simulink model "sampleModel1936_sub_sub_sub"  (R2023a)
settings: Solver=VariableStepAuto  StartTime=0.0  StopTime=10.0  RelTol=1e-3
libraries: hdlsllib x7
settings Model: Creator=user1  LastModifiedBy=user1
settings OptimizationCC: BlockReduction=off  ConditionallyExecuteInputs=off

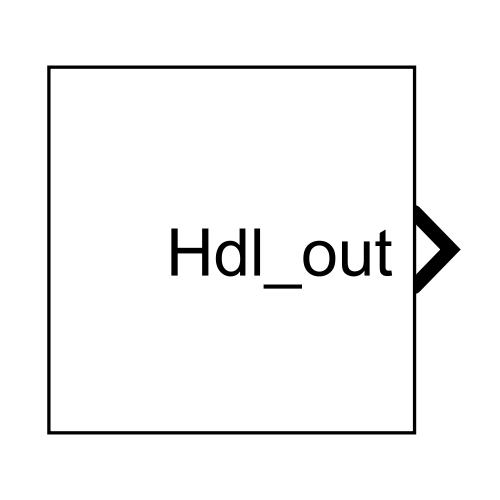
[thumbnail: Simulink's stored preview of the top-level diagram]
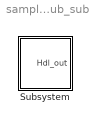
== system sampleModel1936_sub_sub_sub ==
  Subsystem : Subsystem

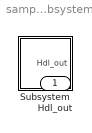
== system sampleModel1936_sub_sub_sub/Subsystem ==
  Subsystem : Subsystem
  Hdl_out : Outport  OutDataTypeStr=uint8

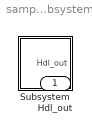
== system sampleModel1936_sub_sub_sub/Subsystem/Subsystem ==
  Subsystem : Subsystem
  Hdl_out : Outport  OutDataTypeStr=uint8

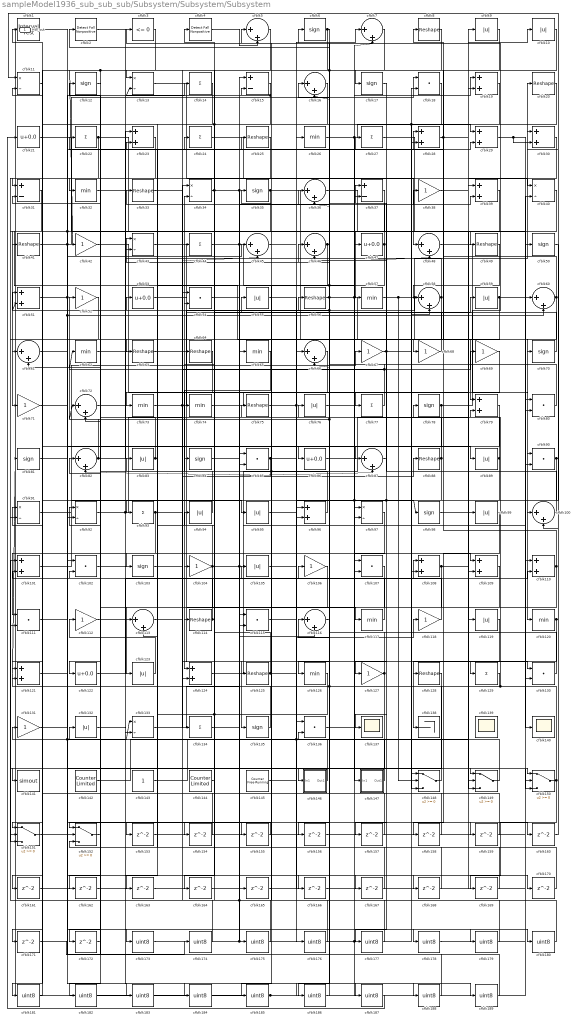
== system sampleModel1936_sub_sub_sub/Subsystem/Subsystem/Subsystem ==
  cfblk1 : hdlsllib/Logic and Bit Operations/Interval Test  IntervalClosedRight=on  uplimit=0.5  IntervalClosedLeft=on  lowlimit=-0.5  OutDataTypeStr=uint8
  cfblk{9..10,55,59,76,83,89,94..95,99,105,119,123,132} (14 alike) : Abs  OutDataTypeStr=uint8  SaturateOnIntegerOverflow=off
  cfblk{5,7,16,36,45..46,48,58,60..61,66,72,82,87,100,113,116} (17 alike) : Sum  Inputs=|++  OutDataTypeStr=uint8
  cfblk{19,23,28..30,39,51,79,96,101,108..110,121,124} (15 alike) : Sum  OutDataTypeStr=uint8
  cfblk{18,54,80,85,90,102,107,111,115,130,136} (11 alike) : DotProduct  OutDataTypeStr=uint8
  cfblk{6,12,17,35,50,70,78,81,84,98,103,135} (12 alike) : Signum
  cfblk{38,42,52,67..69,71,104,106,112,118,127,131} (13 alike) : Gain  OutDataTypeStr=uint8
  cfblk{11,13,34,40,43,91..92,97,133} (9 alike) : Product  Inputs=*/  OutDataTypeStr=uint8  RndMeth=Zero  SaturateOnIntegerOverflow=on
  cfblk{8,20,25,33,41,49,56,63..64,75,88,114,125,128} (14 alike) : Reshape
  cfblk{26,32,57,62,65,73..74,117,120,126} (10 alike) : MinMax  OutDataTypeStr=uint8
  cfblk{21,47,53,86,122} (5 alike) : Bias  Bias=0.0  SaturateOnIntegerOverflow=off
  cfblk{14,22,24,27,44,77,93,129,134} (9 alike) : Sum  Inputs=+  OutDataTypeStr=uint8
  cfblk137 : Scope
  cfblk138 : Terminator
  cfblk139 : Scope
      settings: Floating=on
  cfblk140 : Scope
  cfblk141 : ToWorkspace  VariableName=simout  SaveFormat=Timeseries  SampleTime=-1
  cfblk142 : hdlsllib/Sources/Counter Limited  uplimit=7  tsamp=-1
  cfblk143 : Constant  OutDataTypeStr=uint8  SampleTime=-1
  cfblk144 : hdlsllib/Sources/Counter Limited  uplimit=7  tsamp=-1
  cfblk145 : hdlsllib/Sources/Counter Free-Running  NumBits=16  tsamp=-1
  cfblk146 : Subsystem
      settings: LibrarySourceBlock=|
      | hdlsllib/Ports &
      | Subsystems/Subsystem
  cfblk147 : Subsystem
      settings: LibrarySourceBlock=|
      | hdlsllib/Ports &
      | Subsystems/Subsystem
  cfblk{148..152} (5 alike) : Switch  OutDataTypeStr=uint8  SaturateOnIntegerOverflow=off  InputSameDT=off
  cfblk15 : Sum  Inputs=+-  OutDataTypeStr=uint8
  cfblk{153..172} (20 alike) : Delay  SampleTime=1
  cfblk{173..189} (17 alike) : DataTypeConversion  OutDataTypeStr=uint8  SaturateOnIntegerOverflow=off  RndMeth=Floor
  cfblk2 : hdlsllib/Logic and Bit Operations/Detect Fall Nonpositive  vinit=0  OutDataTypeStr=uint8
  cfblk3 : hdlsllib/Logic and Bit Operations/Compare To Zero  relop=<=  OutDataTypeStr=uint8
  cfblk31 : Sum  Inputs=+-  OutDataTypeStr=uint8
  cfblk37 : Sum  Inputs=+-  OutDataTypeStr=uint8
  cfblk4 : hdlsllib/Logic and Bit Operations/Detect Fall Nonpositive  vinit=0  OutDataTypeStr=uint8
  Hdl_out : Outport  OutDataTypeStr=uint8
  wires:
  cfblk58/1 -> cfblk151/2, cfblk43/1
  cfblk74/1 -> cfblk77/1
  cfblk49/1 -> cfblk55/1
  cfblk78/1 -> cfblk141/1, cfblk6/1
  cfblk150/1 -> cfblk169/1, cfblk79/2, cfblk36/1, cfblk81/1
  cfblk65/1 -> cfblk124/1
  cfblk82/1 -> cfblk25/1, cfblk52/1
  cfblk97/1 -> cfblk103/1
  cfblk41/1 -> cfblk150/1, cfblk18/1
  cfblk31/1 -> cfblk79/1
  cfblk3/1 -> cfblk32/1, cfblk42/1
  cfblk101/1 -> cfblk67/1
  cfblk53/1 -> cfblk135/1
  cfblk88/1 -> cfblk171/1, cfblk53/1
  cfblk108/1 -> cfblk150/2, cfblk123/1
  cfblk70/1 -> cfblk4/1
  cfblk130/1 -> cfblk72/1, cfblk51/2, cfblk36/2
  cfblk7/1 -> cfblk124/2
  cfblk13/1 -> cfblk97/1
  cfblk48/1 -> cfblk120/1
  cfblk9/1 -> cfblk68/1
  cfblk94/1 -> cfblk34/2
  cfblk93/1 -> cfblk88/1, cfblk111/1
  cfblk43/1 -> cfblk117/1
  cfblk5/1 -> cfblk121/1
  cfblk118/1 -> cfblk35/1
  cfblk63/1 -> cfblk59/1
  cfblk125/1 -> cfblk118/1, cfblk24/1
  cfblk26/1 -> cfblk48/2, cfblk29/1
  cfblk33/1 -> cfblk89/1
  cfblk126/1 -> cfblk164/1, cfblk163/1
  cfblk46/1 -> cfblk155/1, cfblk16/1
  cfblk35/1 -> cfblk148/1, cfblk111/2, cfblk92/2
  cfblk51/1 -> cfblk159/1, cfblk14/1
  cfblk83/1 -> cfblk31/2, cfblk113/1
  cfblk56/1 -> cfblk16/2, cfblk7/2, cfblk90/1
  cfblk22/1 -> cfblk91/2, cfblk57/1
  cfblk15/1 -> cfblk181/1, cfblk13/2
  cfblk64/1 -> cfblk73/1
  cfblk40/1 -> cfblk71/1
  cfblk96/1 -> cfblk61/2, cfblk15/2
  cfblk131/1 -> cfblk180/1
  cfblk76/1 -> cfblk109/1
  cfblk129/1 -> cfblk121/2
  cfblk6/1 -> cfblk13/1, cfblk126/1
  cfblk1/1 -> cfblk173/1
  cfblk114/1 -> cfblk12/1, cfblk84/1
  cfblk148/1 -> cfblk51/1, cfblk76/1
  cfblk8/1 -> cfblk17/1
  cfblk66/1 -> cfblk96/2
  cfblk34/1 -> cfblk154/1, cfblk87/2, cfblk29/2
  cfblk47/1 -> cfblk2/1, cfblk63/1, cfblk66/2
  cfblk68/1 -> cfblk5/1
  cfblk30/1 -> cfblk104/1
  cfblk147/1(Out1) -> cfblk136/2
  cfblk90/1 -> cfblk177/1, cfblk11/1
  cfblk80/1 -> cfblk33/1
  cfblk98/1 -> cfblk109/2
  cfblk115/1 -> cfblk108/1
  cfblk133/1 -> cfblk65/1
  cfblk24/1 -> cfblk48/1
  cfblk87/1 -> cfblk37/1
  cfblk59/1 -> cfblk87/1, cfblk60/1
  cfblk127/1 -> cfblk151/3, cfblk3/1
  cfblk73/1 -> cfblk45/2, cfblk20/1
  cfblk142/1 -> cfblk9/1
  cfblk21/1 -> cfblk110/1
  cfblk79/1 -> cfblk113/2
  cfblk62/1 -> cfblk134/1
  cfblk20/1 -> cfblk127/1
  cfblk28/1 -> cfblk58/1, cfblk10/1
  cfblk39/1 -> cfblk122/1
  cfblk89/1 -> cfblk75/1, cfblk115/2, cfblk137/1
  cfblk135/1 -> cfblk82/1
  cfblk60/1 -> cfblk70/1, cfblk22/1
  cfblk95/1 -> cfblk149/1
  cfblk110/1 -> cfblk156/1, cfblk8/1
  cfblk103/1 -> cfblk129/1
  cfblk50/1 -> cfblk100/1
  cfblk120/1 -> cfblk149/3, cfblk30/1
  cfblk117/1 -> cfblk11/2
  cfblk71/1 -> cfblk85/2
  cfblk143/1 -> cfblk28/2, cfblk26/1
  cfblk122/1 -> cfblk110/2
  cfblk119/1 -> cfblk138/1
  cfblk72/1 -> cfblk23/1
  cfblk23/1 -> cfblk152/2
  cfblk11/1 -> cfblk31/1
  cfblk151/1 -> cfblk133/1, cfblk27/1
  cfblk146/1(Out1) -> cfblk91/1
  cfblk29/1 -> cfblk30/2, cfblk140/1
  cfblk136/1 -> cfblk19/1
  cfblk45/1 -> cfblk7/1
  cfblk57/1 -> cfblk148/2, cfblk40/2, cfblk119/1
  cfblk37/1 -> cfblk146/1(In1)
  cfblk67/1 -> cfblk37/2, cfblk130/1
  cfblk144/1 -> cfblk64/1
  cfblk124/1 -> cfblk39/1
  cfblk27/1 -> cfblk99/1
  cfblk84/1 -> cfblk116/2
  cfblk123/1 -> cfblk112/1
  cfblk36/1 -> cfblk49/1
  cfblk100/1 -> cfblk46/2
  cfblk14/1 -> cfblk41/1
  cfblk19/1 -> cfblk108/2, cfblk151/1, cfblk114/1
  cfblk85/1 -> cfblk28/1, cfblk82/2
  cfblk44/1 -> cfblk39/2, cfblk147/1(In1)
  cfblk91/1 -> cfblk95/1
  cfblk99/1 -> cfblk128/1
  cfblk4/1 -> cfblk5/2
  cfblk111/1 -> cfblk60/2, cfblk45/1
  cfblk86/1 -> cfblk78/1
  cfblk75/1 -> cfblk38/1, cfblk97/2, cfblk98/1
  cfblk152/1 -> cfblk92/1
  cfblk113/1 -> cfblk69/1
  cfblk18/1 -> cfblk61/1
  cfblk92/1 -> cfblk150/3, cfblk44/1
  cfblk38/1 -> cfblk40/1
  cfblk104/1 -> cfblk133/2, cfblk83/1, cfblk148/3, cfblk50/1
  cfblk77/1 -> cfblk43/2, cfblk62/1
  cfblk10/1 -> cfblk74/1, cfblk86/1
  cfblk116/1 -> cfblk56/1
  cfblk42/1 -> cfblk149/2
  cfblk16/1 -> cfblk93/1
  cfblk149/1 -> cfblk132/1
  cfblk69/1 -> cfblk153/1
  cfblk153/1 -> cfblk90/2
  cfblk154/1 -> cfblk101/2
  cfblk155/1 -> cfblk152/1
  cfblk156/1 -> cfblk46/1
  cfblk17/1 -> cfblk157/1
  cfblk157/1 -> cfblk34/1
  cfblk109/1 -> cfblk158/1
  cfblk158/1 -> cfblk15/1
  cfblk159/1 -> cfblk136/1
  cfblk121/1 -> cfblk160/1
  cfblk160/1 -> cfblk100/2
  cfblk52/1 -> cfblk161/1
  cfblk161/1 -> cfblk85/1
  cfblk25/1 -> cfblk162/1
  cfblk163/1 -> cfblk66/1
  cfblk164/1 -> cfblk130/2
  cfblk134/1 -> cfblk165/1
  cfblk165/1 -> cfblk19/2
  cfblk112/1 -> cfblk166/1
  cfblk166/1 -> cfblk18/2
  cfblk81/1 -> cfblk167/1
  cfblk167/1 -> cfblk152/3
  cfblk55/1 -> cfblk168/1
  cfblk168/1 -> cfblk116/1
  cfblk169/1 -> cfblk23/2
  cfblk132/1 -> cfblk170/1
  cfblk170/1 -> cfblk96/1
  cfblk12/1 -> cfblk172/1
  cfblk172/1 -> cfblk72/2
  cfblk173/1 -> cfblk125/1, cfblk47/1, cfblk58/2
  cfblk171/1 -> cfblk174/1
  cfblk174/1 -> cfblk1/1
  cfblk54/1 -> cfblk175/1
  cfblk175/1 -> cfblk94/1
  cfblk145/1 -> cfblk176/1
  cfblk176/1 -> cfblk54/1
  cfblk177/1 -> cfblk54/2
  cfblk105/1 -> cfblk178/1
  cfblk178/1 -> cfblk80/2
  cfblk32/1 -> cfblk179/1
  cfblk179/1 -> cfblk105/1
  cfblk180/1 -> cfblk101/1, cfblk115/1
  cfblk181/1 -> cfblk131/1
  cfblk107/1 -> cfblk182/1
  cfblk182/1 -> cfblk80/1
  cfblk61/1 -> cfblk183/1
  cfblk183/1 -> cfblk107/1
  cfblk162/1 -> cfblk184/1
  cfblk184/1 -> cfblk107/2
  cfblk106/1 -> cfblk185/1
  cfblk128/1 -> cfblk186/1
  cfblk186/1 -> cfblk106/1
  cfblk102/1 -> cfblk187/1
  cfblk187/1 -> cfblk21/1
  cfblk185/1 -> Hdl_out/1, cfblk188/1
  cfblk188/1 -> cfblk102/1
  cfblk2/1 -> cfblk189/1
  cfblk189/1 -> cfblk102/2

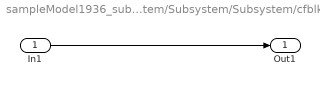
== system sampleModel1936_sub_sub_sub/Subsystem/Subsystem/Subsystem/cfblk146 ==
  In1 : Inport
  Out1 : Outport
  wires:
  In1/1 -> Out1/1

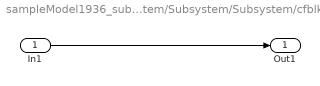
== system sampleModel1936_sub_sub_sub/Subsystem/Subsystem/Subsystem/cfblk147 ==
  In1 : Inport
  Out1 : Outport
  wires:
  In1/1 -> Out1/1
